simulink model "MotionReference"  (R2023b)
settings: Solver=FixedStepAuto  StartTime=0.0  StopTime=25  FixedStep=0.01  RelTol=1e-3
settings Model: Creator=Jakob  LastModifiedBy=Jakob

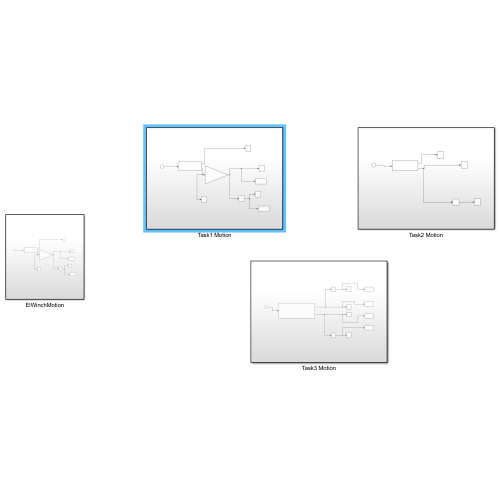
[thumbnail: Simulink's stored preview of the top-level diagram]
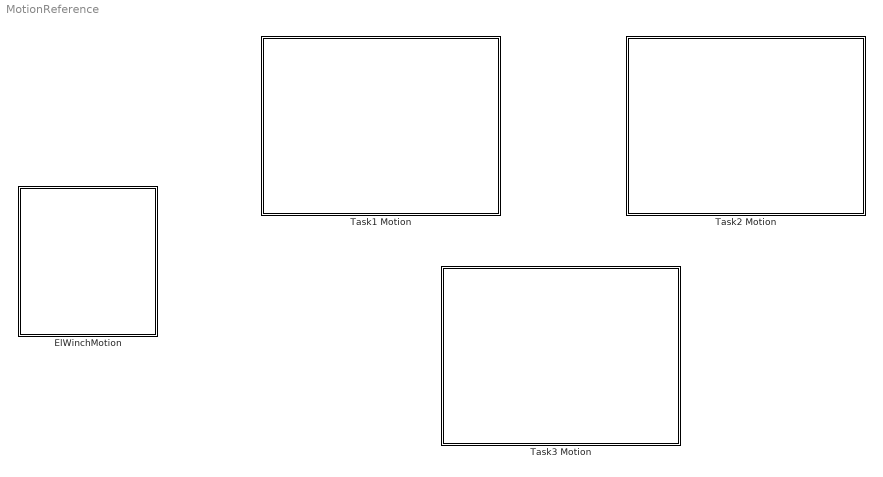
== system MotionReference ==
  ElWinchMotion : Subsystem
  Task1 Motion : Subsystem
  Task2 Motion : Subsystem
  Task3 Motion : Subsystem

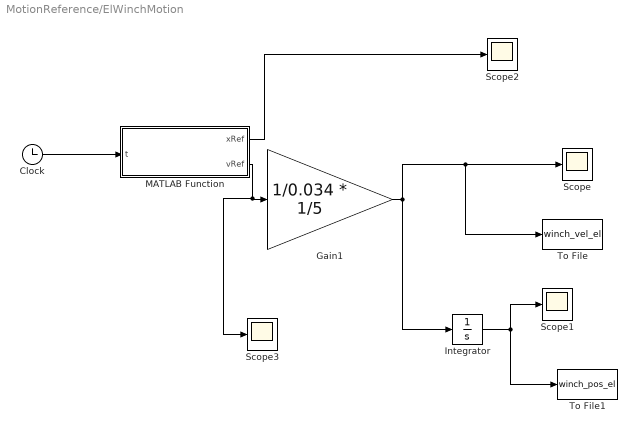
== system MotionReference/ElWinchMotion ==
  Clock : Clock
  Gain1 : Gain  Gain=1/0.034 * 1/5
  Integrator : Integrator
  MATLAB Function : MATLAB Function  TreatAsAtomicUnit=on
  Scope{,1..3} (4 alike) : Scope
  To File : ToFile  Filename=winch_vel_el  MatrixName=winch_vel  SaveFormat=Timeseries  SampleTime=0.01
      settings: Decimation=2
  To File1 : ToFile  Filename=winch_pos_el  MatrixName=winch_pos  SaveFormat=Timeseries  SampleTime=0.01
      settings: Decimation=2
  wires:
  Integrator/1 -> To File1/1, Scope1/1
  MATLAB Function/2(vRef) -> Scope3/1, Gain1/1
  Clock/1 -> MATLAB Function/1(t)
  MATLAB Function/1(xRef) -> Scope2/1
  Gain1/1 -> To File/1, Scope/1, Integrator/1

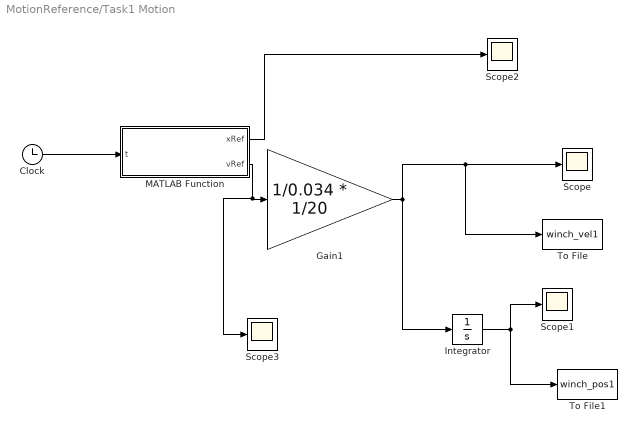
== system MotionReference/Task1 Motion ==
  Clock : Clock
  Gain1 : Gain  Gain=1/0.034 * 1/20
  Integrator : Integrator
  MATLAB Function : MATLAB Function  TreatAsAtomicUnit=on
  Scope{,1..3} (4 alike) : Scope
  To File : ToFile  Filename=winch_vel1  MatrixName=winch_vel  SaveFormat=Timeseries  SampleTime=0.01
      settings: Decimation=2
  To File1 : ToFile  Filename=winch_pos1  MatrixName=winch_pos  SaveFormat=Timeseries  SampleTime=0.01
      settings: Decimation=2
  wires:
  Integrator/1 -> To File1/1, Scope1/1
  Clock/1 -> MATLAB Function/1(t)
  MATLAB Function/1(xRef) -> Scope2/1
  MATLAB Function/2(vRef) -> Scope3/1, Gain1/1
  Gain1/1 -> To File/1, Scope/1, Integrator/1

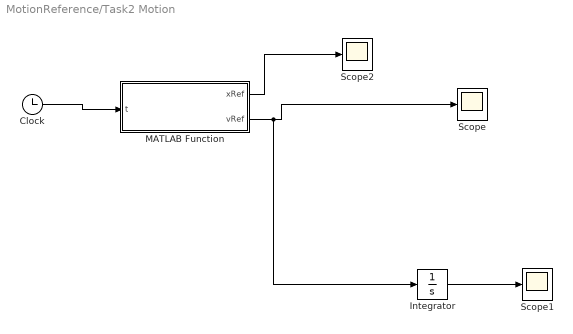
== system MotionReference/Task2 Motion ==
  Clock : Clock
  Integrator : Integrator  InitialCondition=0.05
  MATLAB Function : MATLAB Function  TreatAsAtomicUnit=on
  Scope : Scope
  Scope1 : Scope
  Scope2 : Scope
  wires:
  Integrator/1 -> Scope1/1
  MATLAB Function/2(vRef) -> Integrator/1, Scope/1
  Clock/1 -> MATLAB Function/1(t)
  MATLAB Function/1(xRef) -> Scope2/1

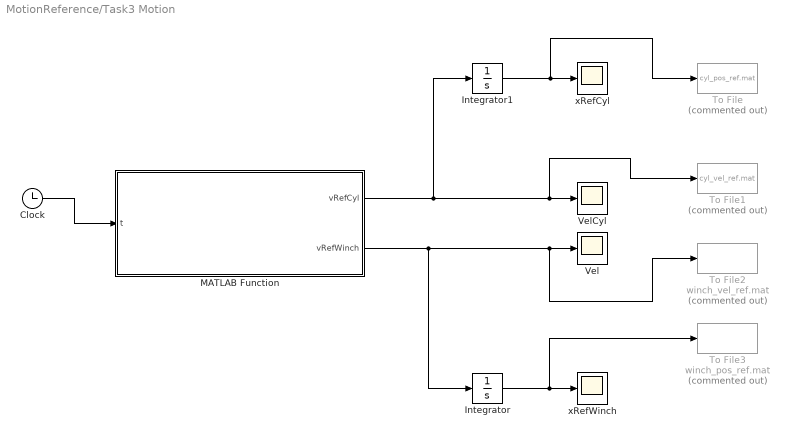
== system MotionReference/Task3 Motion ==
  Clock : Clock
  Integrator : Integrator  InitialCondition=0.1
  Integrator1 : Integrator  InitialCondition=0.05
  MATLAB Function : MATLAB Function  TreatAsAtomicUnit=on
  To File : ToFile  Commented=on  Filename=cyl_pos_ref.mat  MatrixName=cyl_pos_task3  SaveFormat=Timeseries
  To File1 : ToFile  Commented=on  Filename=cyl_vel_ref.mat  MatrixName=cyl_vel_task3  SaveFormat=Timeseries
  To File2 : ToFile  Commented=on  Filename=winch_vel_ref.mat  MatrixName=winch_vel_task3  SaveFormat=Timeseries
  To File3 : ToFile  Commented=on  Filename=winch_pos_ref.mat  MatrixName=winch_pos_task3  SaveFormat=Timeseries
  Vel : Scope
  VelCyl : Scope
  xRefCyl : Scope
  xRefWinch : Scope
  wires:
  Integrator/1 -> To File3/1, xRefWinch/1
  MATLAB Function/2(vRefWinch) -> To File2/1, Vel/1, Integrator/1
  Clock/1 -> MATLAB Function/1(t)
  MATLAB Function/1(vRefCyl) -> Integrator1/1, To File1/1, VelCyl/1
  Integrator1/1 -> To File/1, xRefCyl/1

== matlab function MotionReference/Task1 Motion/MATLAB Function ==
  data: xRef output; t input; vRef output
function [xRef,vRef] = MotionRefTask1(t)
xRef = 0.1;

vRef = 0.0;

tRamp = 1.0;

vSet = 0.039;
if t < 1.0
    vRef = 0.0;
elseif t >= 1.0 && t < 2.0
    vRef = vSet*(t - tRamp);
elseif t >= 2.0 && t < 8.0
    vRef = vSet;
elseif t >= 8.0 && t < 9.0
    t1 = (t - 9.0);
    vRef = -vSet * t1;
elseif t >=9.0 && t < 14.0
    vRef = 0.0; 
elseif t >=14.0 && t < 15.0
    t2 = (t - 14.0);
    vRef = -vSet * t2;
elseif t >= 15.0 && t < 21.0
    vRef = -vSet;
elseif t >= 21.0 && t < 22.0
    t3 = t - 21.0;
    vRef = vSet * t3 - vSet;
end 


end

== matlab function MotionReference/Task3 Motion/MATLAB Function ==
  data: vRefCyl output; t input; vRefWinch output
function [vRefCyl,vRefWinch] = MotionRefTask1(t)
xRef = 0.1;

vRefCyl = 0.0;
vRefWinch = 0.0; 

tRamp = 1.0;

vSetWinch = 0.071;
vSetCyl = 0.05;

if t < 1.0
    vRefWinch = 0.0;
    vRefCyl = 0.0;
elseif t >= 1.0 && t < 2.0
    vRefWinch = vSetWinch*(t - tRamp);
    vRefCyl = 0.0;
elseif t >= 2.0 && t < 8.0
    vRefWinch = vSetWinch;
    vRefCyl = 0.0;
elseif t >= 8.0 && t < 9.0
    t1 = (t - 8.0);
    vRefWinch = -vSetWinch * t1 + vSetWinch;
    vRefCyl = 0.0;
elseif t >=9.0 && t < 10.0
    vRefWinch = 0.0; 
    vRefCyl = 0.0;

elseif t >=11.0 && t < 12.0
    t2 = (t - 11.0);
    vRefCyl = vSetCyl * t2;
    vRefWinch = 0.0; 
elseif t >= 12.0 && t < 19.0
    vRefCyl = vSetCyl;
    vRefWinch = 0.0; 
elseif t >= 19.0 && t < 20.0
    t3 = t - 19.0;
    vRefCyl = -vSetCyl * t3 + vSetCyl;
    vRefWinch = 0.0; 
elseif t >=20.0 && t < 25.0
    vRefCyl = 0.0; 
    vRefWinch = 0.0; 
elseif t >= 25.0 && t < 26.0
    t4 = t - 25.0;
    vRefCyl = -vSetCyl*t4;
    vRefWinch = 0.0; 
elseif t >= 26.0 && t < 33.0
    vRefCyl = -vSetCyl; 
    vRefWinch = 0.0; 
elseif t >= 33.0 && t < 34.0
    t5 = t - 33.0;
    vRefCyl = vSetCyl * t5 - vSetCyl; 
    vRefWinch = 0.0; 
elseif t >= 39.0 && t < 40.0
    t6 = t - 39.0;
    vRefWinch = -vSetWinch * t6;
    vRefCyl = 0.0;
elseif t >= 40.0 && t < 46.0
    vRefWinch = -vSetWinch;
    vRefCyl = 0.0;
elseif t >= 46.0 && t < 47.0
    t7 = t - 46.0;
    vRefWinch = vSetWinch*t7 - vSetWinch;
    vRefCyl = 0.0; 
end 


end

== matlab function MotionReference/ElWinchMotion/MATLAB Function ==
  data: xRef output; t input; vRef output
function [xRef,vRef] = MotionRefTask1(t)
xRef = 0.1;

vRef = 0.0;

tRamp = 1.0;

vSet = 1.0;
if t < 1.0
    vRef = 0.0;
elseif t >= 1.0 && t < 2.0
    vRef = vSet*(t - tRamp);
elseif t >= 2.0 && t < 8.0
    vRef = vSet;
elseif t >= 8.0 && t < 9.0
    t1 = (t - 9.0);
    vRef = -vSet * t1;
elseif t >=9.0 && t < 14.0
    vRef = 0.0; 
elseif t >=14.0 && t < 15.0
    t2 = (t - 14.0);
    vRef = -vSet * t2;
elseif t >= 15.0 && t < 21.0
    vRef = -vSet;
elseif t >= 21.0 && t < 22.0
    t3 = t - 21.0;
    vRef = vSet * t3 - vSet;
end 


end

== matlab function MotionReference/Task2 Motion/MATLAB Function ==
  data: xRef output; t input; vRef output
function [xRef,vRef] = MotionRefTask1(t)
xRef = 0.1;

vRef = 0.0;

tRamp = 1.0;

vSet = 0.05;
if t < 1.0
    vRef = 0.0;
elseif t >= 1.0 && t < 2.0
    vRef = vSet*(t - tRamp);
elseif t >= 2.0 && t < 9.0
    vRef = vSet;
elseif t >= 9.0 && t < 10.0
    t1 = (t - 9.0);
    vRef = -vSet * t1 + 0.05;
elseif t >=9.0 && t < 14.0
    vRef = 0.0; 
elseif t >=15.0 && t < 16.0
    t2 = (t - 15.0);
    vRef = -vSet * t2;
elseif t >= 15.0 && t < 23.0
    vRef = -vSet;
elseif t >= 23.0 && t < 24.0
    t3 = t - 23.0;
    vRef = vSet * t3 - vSet;
end 


end
